simulink model "labONE"  (R2023b)
settings: Solver=VariableStepAuto  StartTime=0.0  StopTime=10  RelTol=1e-3
libraries: dspfdesign x1, dspsrcs4 x1
settings Model: Creator=omarf  LastModifiedBy=omarf

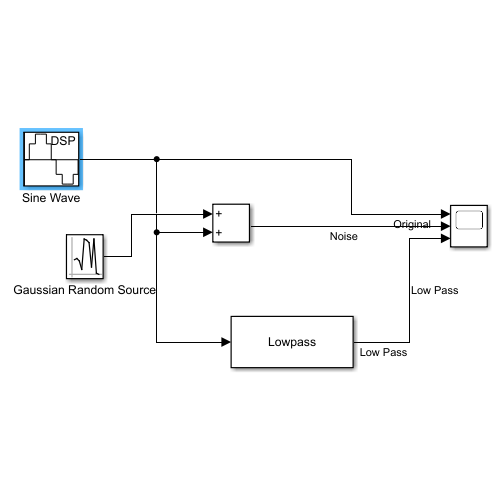
[thumbnail: Simulink's stored preview of the top-level diagram]
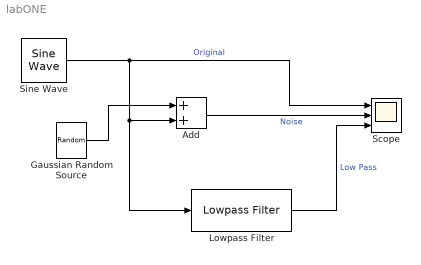
== system labONE ==
  Add : Sum
  Gaussian Random Source : RandomNumber  SampleTime=0.1
  Lowpass Filter : dspfdesign/Lowpass Filter  FilterType=FIR  DesignForMinimumOrder=on  FilterOrder=50  PassbandFrequency=2  StopbandFrequency=5  PassbandRipple=1  StopbandAttenuation=60  SampleRateMode=Specify on dialog  SampleRate=100  SimulateUsing=Interpreted execution  roundingMode=Floor  coeffsDataTypeStr=fixdt(1,16)
  Scope : Scope  NumInputPorts=3
  Sine Wave : dspsrcs4/Sine Wave  Amplitude=5  Frequency=1  Phase=0  SampleMode=Discrete  OutComplex=Real  CompMethod=Trigonometric fcn  TableSize=Speed  SampleTime=0.01  SamplesPerFrame=1  ResetState=Restart at time zero  OutputFrames=off  dataType=double  wordLen=16  udDataType=sfix(16)  fracBitsMode=Best precision  numFracBits=15  OutDataTypeStr=double  LastOutDataTypeStr=double
  wires:
  Lowpass Filter/1 -> Scope/3  "Low Pass"
  Sine Wave/1 -> Lowpass Filter/1, Add/2, Scope/1  "Original"
  Add/1 -> Scope/2  "Noise"
  Gaussian Random Source/1 -> Add/1
